simulink model "modelLab4"  (R2023a)
settings: Solver=VariableStepAuto  StartTime=0.0  StopTime=20  RelTol=1e-3
values from neighbouring files (symbols this model uses):
  A = [0, 1 ... (first row only)    [initHW4.m]    (also in initLab4.m = [0, 1, 0, 0; lab5m.m = [-f1 0;f1 -f2])
  Ao = phi - L * C - gamma * K    [initLab4.m]
  B = [0 ... (first row only)    [initHW4.m]    (also in initLab4.m = [0; (constA .* constD)./(n .* g); 0; constD]; lab5m.m = [beta;0])
  Bo = L    [initLab4.m]
  C = [1, 0]    [initHW4.m]    (also in initLab4.m = [1, 0, 0, 0; lab5m.m = [0 1])
  Co = -K    [initLab4.m]
  D = 0    [initHW4.m]    (also in initLab4.m = zeros(2,1))
  Do = zeros(1,2)    [initLab4.m]
  q = 10 ^ (UGM / 20)    (= 1.01741936618)    [initLab4.m]
  T = min(Ts / 20 * (nOrder + 1),      pi / (5 * TbetaMax))    [initHW4.m]    (also in initLab4.m = 0.01; lab5m.m = 0.1)
  x0 = [0.17; 0; 0; 0]    [initLab4.m]
  xo0 = C \ (C * x0)    [initLab4.m]
settings Model: Creator=fwah  LastModifiedBy=fwah
settings OptimizationCC: ReuseModelBlockBuffer=off

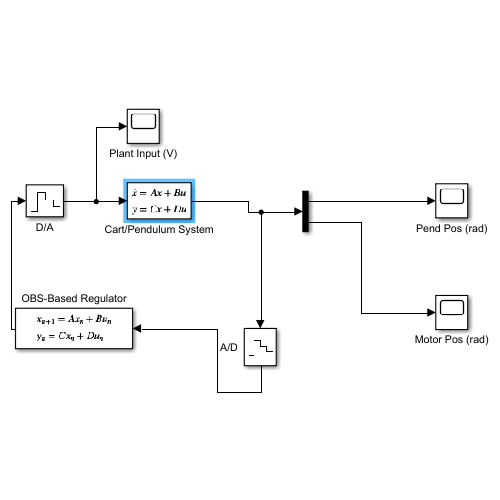
[thumbnail: Simulink's stored preview of the top-level diagram]
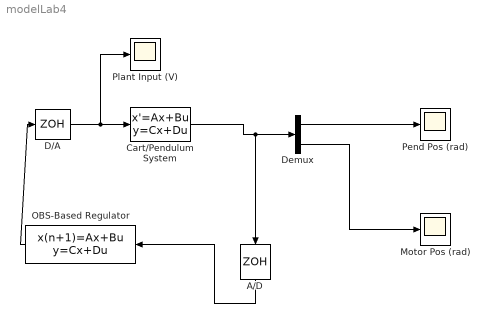
== system modelLab4 ==
  A/D : ZeroOrderHold  SampleTime=T
  Cart/Pendulum System : StateSpace  A=A  B=q * B  C=C  D=D  InitialCondition=x0
  D/A : ZeroOrderHold  SampleTime=T
  Demux : Demux  Outputs=2
  Motor Pos (rad) : Scope
  OBS-Based Regulator : DiscreteStateSpace  A=Ao  B=Bo  C=Co  D=Do  InitialCondition=xo0  SampleTime=T
  Pend Pos (rad) : Scope
  Plant Input (V) : Scope
  wires:
  D/A/1 -> Cart/Pendulum System/1, Plant Input (V)/1
  Demux/1 -> Pend Pos (rad)/1
  Demux/2 -> Motor Pos (rad)/1
  Cart/Pendulum System/1 -> A/D/1, Demux/1
  A/D/1 -> OBS-Based Regulator/1
  OBS-Based Regulator/1 -> D/A/1
